simulink model "Planta_Funcional_17_03_24"  (R2021a)
settings: Solver=VariableStepAuto  StartTime=0.0  StopTime=120  MaxStep=1e-2  RelTol=1e-3
values from neighbouring files (symbols this model uses):
  ahmax = 0.75    [valoresPlanta_29_9_24.m]    (also in valoresPlanta_V3.m)
  alfahmax = ((2*ahmax)/(rhd))    (= 2)    [valoresPlanta_29_9_24.m]    (also in valoresPlanta_V3.m)
  alfatmax = atmax/rtd    (= 1.6)    [valoresPlanta_29_9_24.m]    (also in valoresPlanta_V3.m)
  atmax = 0.8    [valoresPlanta_29_9_24.m]    (also in valoresPlanta_V3.m)
  ax_max = 0.8    [valoresPlanta_29_9_24.m]    (also in valoresPlanta_v4.m)
  ay_max = 0.75    [valoresPlanta_29_9_24.m]    (also in valoresPlanta_v4.m)
  bcx = 1e6    (= 1000000)    [Valores_1.m]    (also in valoresPlanta.m; valoresPlanta_29_9_24.m; valoresPlanta_V3.m; valoresPlanta_v4.m)
  bcy = 1e7    (= 10000000)    [Valores_1.m]    (also in valoresPlanta.m; valoresPlanta_29_9_24.m; valoresPlanta_V3.m; valoresPlanta_v4.m)
  bh_eq = bhm*ih^2+bhd    (= 8720)    [Valores.m]    (also in Valores_1.m; valoresPlanta.m; valoresPlanta_29_9_24.m; valoresPlanta_V3.m)
  bhb = 1e8    (= 100000000)    [Valores.m]    (also in Valores_1.m; valoresPlanta.m; valoresPlanta_29_9_24.m; valoresPlanta_V3.m)
  bhEb = 2.2e9    (= 2200000000)    [Valores.m]    (also in Valores_1.m; valoresPlanta.m; valoresPlanta_29_9_24.m; valoresPlanta_V3.m)
  bt = 90.0    (= 90)    [Valores.m]    (also in Valores_1.m; valoresPlanta.m; valoresPlanta_29_9_24.m; valoresPlanta_V3.m)
  bt_eq = btd+(btm*(it^2))    (= 5401.8)    [valoresPlanta.m]    (also in valoresPlanta_29_9_24.m; valoresPlanta_V3.m; valoresPlanta_v4.m)
  btb = 5e6    (= 5000000)    [Valores.m]    (also in Valores_1.m; valoresPlanta.m; valoresPlanta_29_9_24.m; valoresPlanta_V3.m)
  btw = 3.0e3    (= 3000)    [Valores.m]    (also in Valores_1.m; valoresPlanta.m; valoresPlanta_29_9_24.m; valoresPlanta_V3.m)
  bwu = 150    [Valores.m]    (also in Valores_1.m; valoresPlanta.m; valoresPlanta_29_9_24.m; valoresPlanta_V3.m)
  estado_cont = [x_positions; hy_cont]    [perfilObsaculos.m]    (also in valoresPlanta_29_9_24.m = [x_positions; [hy_muelle hy_cont]])
  g = 9.80665    [Valores.m]    (also in Valores_1.m; valoresPlanta.m; valoresPlanta_29_9_24.m; valoresPlanta_V3.m)
  Hc = 0    [Valores.m]    (also in Valores_1.m = 2.5; valoresPlanta.m = 2.5; valoresPlanta_29_9_24.m = 2.5; valoresPlanta_V3.m = 2.5)
  hx_cont = 2.5    [perfilObsaculos.m]    (also in puntosTrayectoria.m; valoresPlanta_29_9_24.m)
  ih = 22    [Valores.m]    (also in Valores_1.m; valoresPlanta.m; valoresPlanta_29_9_24.m; valoresPlanta_V3.m)
  it = 30    [Valores.m]    (also in Valores_1.m; valoresPlanta.m; valoresPlanta_29_9_24.m; valoresPlanta_V3.m)
  Jh_eq = Jhm_hb*ih^2+Jhd_hEb    (= 18320)    [Valores.m]    (also in Valores_1.m; valoresPlanta.m; valoresPlanta_29_9_24.m; valoresPlanta_V3.m)
  Jt_eq = Jtd+(Jtm_tb*(it^2))    (= 7500)    [valoresPlanta.m]    (also in valoresPlanta_29_9_24.m; valoresPlanta_V3.m; valoresPlanta_v4.m)
  kcy = 1.8e9    (= 1800000000)    [Valores_1.m]    (also in valoresPlanta.m; valoresPlanta_29_9_24.m; valoresPlanta_V3.m; valoresPlanta_v4.m)
  KDh = Jeq2 * w_posh^3    (= -12245.4404091)    [Valores.m]    (also in Valores_1.m = Jeq2 * w_posh; valoresPlanta.m = Jeq2 * w_posh; valoresPlanta_29_9_24.m = Jh_eq * n * w_posh; valoresPlanta_V3.m = Jeq2 * w_posh)
  KDt = Meq2 * w_post^3    (= -4728.86946035)    [Valores.m]    (also in Valores_1.m = Meq2 * w_post; valoresPlanta.m = Meq2 * w_post; valoresPlanta_29_9_24.m = 10127; valoresPlanta_V3.m = Meq2 * w_post)
  KIh = Jeq2 * w_posh^2    (= 2572.66592082)    [Valores.m]    (also in Valores_1.m = Jeq2 * w_posh^3; valoresPlanta.m = Jeq2 * w_posh^3; valoresPlanta_29_9_24.m = Jh_eq * w_posh^3; valoresPlanta_V3.m = Jeq2 * w_posh^3)
  KIt = Meq2 * w_post^2    (= 1307.690244)    [Valores.m]    (also in Valores_1.m = Meq2 * w_post^3; valoresPlanta.m = Meq2 * w_post^3; valoresPlanta_29_9_24.m = 6809.6; valoresPlanta_V3.m = Meq2 * w_post^3)
  KPh = Jeq2 * w_posh    (= -540.495867769)    [Valores.m]    (also in Valores_1.m = Jeq2 * w_posh^2; valoresPlanta.m = Jeq2 * w_posh^2; valoresPlanta_29_9_24.m = Jh_eq * n * w_posh^2; valoresPlanta_V3.m = Jeq2 * w_posh^2)
  KPt = Meq2 * w_post    (= -361.62)    [Valores.m]    (also in Valores_1.m = Meq2 * w_post^2; valoresPlanta.m = Meq2 * w_post^2; valoresPlanta_29_9_24.m = 14123; valoresPlanta_V3.m = Meq2 * w_post^2)
  Ktw = 4.8e5    (= 480000)    [Valores.m]    (also in Valores_1.m; valoresPlanta.m; valoresPlanta_29_9_24.m; valoresPlanta_V3.m)
  kwu = 2.36e8    (= 236000000)    [Valores.m]    (also in Valores_1.m; valoresPlanta.m; valoresPlanta_29_9_24.m; valoresPlanta_V3.m)
  Mc_max = 5e4    (= 50000)    [Valores.m]    (also in Valores_1.m; valoresPlanta.m; valoresPlanta_29_9_24.m; valoresPlanta_V3.m)
  Mc_min = 2e3    (= 2000)    [Valores.m]    (also in Valores_1.m; valoresPlanta.m; valoresPlanta_29_9_24.m; valoresPlanta_V3.m)
  Meq = Mt+(it^2*Jtm_tb+Jtd)/rtd^2    (= 60000)    [Valores.m]    (also in Valores_1.m; valoresPlanta_29_9_24.m; valoresPlanta_v4.m)
  Mt = 30000    [Valores.m]    (also in Valores_1.m; valoresPlanta.m; valoresPlanta_29_9_24.m; valoresPlanta_V3.m)
  pos = [p0; p1; p2; p3; p4; p5]    [calcularTrayectoria2_prueba.m]    (also in perfilObsaculos.m = puntosTrayectoria(4, 1.5, 20, [-20,0], estado_cont, hy_cont,; puntosTrayectoria.m; valoresPlanta_29_9_24.m = calcularTrayectoria2_prueba(vx_max, vhmax, ax_max, Hc, hx_co)
  rhd = 0.75    [Valores.m]    (also in Valores_1.m; valoresPlanta.m; valoresPlanta_29_9_24.m; valoresPlanta_V3.m)
  rtd = 0.5    [Valores.m]    (also in Valores_1.m; valoresPlanta.m; valoresPlanta_29_9_24.m; valoresPlanta_V3.m)
  tau_hm = 1e-3    (= 0.001)    [valoresPlanta.m]    (also in valoresPlanta_29_9_24.m; valoresPlanta_V3.m; valoresPlanta_v4.m)
  tau_tm = 1e-3    (= 0.001)    [Valores.m]    (also in Valores_1.m; valoresPlanta.m; valoresPlanta_29_9_24.m; valoresPlanta_V3.m)
  Thb_Max = 5e4    (= 50000)    [Valores.m]    (also in Valores_1.m; valoresPlanta.m; valoresPlanta_29_9_24.m; valoresPlanta_V3.m)
  ThEb_Max = 1.1e6    (= 1100000)    [Valores.m]    (also in Valores_1.m; valoresPlanta.m; valoresPlanta_29_9_24.m; valoresPlanta_V3.m)
  Thm_Max = 2e4    (= 20000)    [Valores.m]    (also in Valores_1.m; valoresPlanta.m; valoresPlanta_29_9_24.m; valoresPlanta_V3.m)
  Ttb_Max = 5e3    (= 5000)    [Valores.m]    (also in Valores_1.m; valoresPlanta.m; valoresPlanta_29_9_24.m; valoresPlanta_V3.m)
  Ttm_Max = 3e3    (= 3000)    [Valores.m]    (also in Valores_1.m; valoresPlanta.m; valoresPlanta_29_9_24.m = 4000; valoresPlanta_V3.m)
  v_x_max = 4    [Valores_1.m]    (also in valoresPlanta.m; valoresPlanta_V3.m = 0.4; valoresPlanta_v4.m)
  vhmax = 3    [valoresPlanta_29_9_24.m]    (also in valoresPlanta_V3.m)
  vx_max = 4    [valoresPlanta_29_9_24.m]
  whmMax = P/Thm_Max    (= 47.8075)    [Valores_1.m]    (also in valoresPlanta.m; valoresPlanta_29_9_24.m = 176; valoresPlanta_V3.m; valoresPlanta_v4.m)
  wtmMax = (4/rtd)*it    (= 240)    [Valores_1.m]    (also in valoresPlanta.m; valoresPlanta_29_9_24.m; valoresPlanta_V3.m; valoresPlanta_v4.m)
  y0 = 2.5    [valoresPlanta_29_9_24.m]
  Yt0 = 45    [Valores.m]    (also in Valores_1.m; valoresPlanta.m; valoresPlanta_29_9_24.m; valoresPlanta_V3.m)
undefined symbols (not defined in the file or in its folder): sigbuilder_block, x0
libraries: vrlib x2, simulink_extras x1, aerolibanimutils x1, cstblocks x1, simulink x1
(part 1 of 2)
settings Model: Creator=Matias  LastModifiedBy=Matias

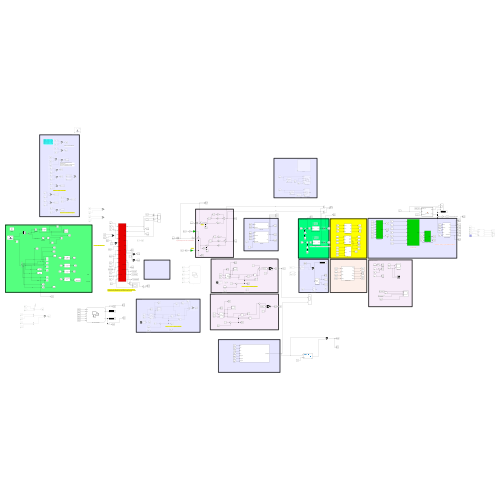
[thumbnail: Simulink's stored preview of the top-level diagram]
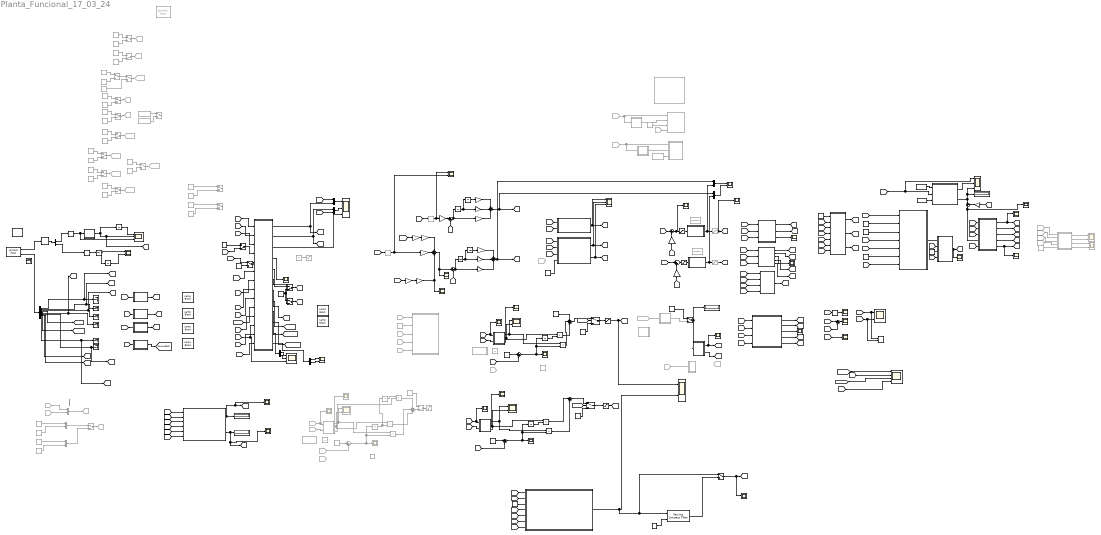
== system Planta_Funcional_17_03_24 ==
  note: Aca hacer la estimacion de masa
  note: Corregir con nivel 0 el estado de emergencia
  note: Estimación de carga: subir la carga lento (cuasiestático) y una vez que el cable esté completamente elongado determinar la masa. Se puede calcular para cierta velocidad cuanto debo demorar y darle ese tiempo para calcular la masa con la Fhw.
  note: FRENOS: 0 activados, 1 desactivados
  note: Frenos
  note: saturador a la salida?? o a la entrada de consigna de torque??
  note: Indicadores
  note: ciclo=0 y to_where=0 --> a barco
      | ciclo=0 y to_where=1 --> a muelle
      | -------------------------------------------------
      | ciclo=1 y to_where=0 --> a barco
      | ciclo=1 y to_where=1 --> a barco 2
      | ciclo=1 y to_where=2 --> a muelle
  note: revisar para modo manual
  note: ec2 cable tensado
  note: PI balanceo
  note: con ganancia baja, si sumo o resto no hace diferencia
  note: Control P
  note: por que v y no theta? no cambian las ganancias?
  note: d(theta)/dt
  note: Analisis de posiciones
  note: PD Balanceo
  note: Masa Variable
  note: Control Frenos
  note: Izaje
  note: Modulador de Torque
  note: Carro
  note: Movimiento
  note: PID Balanceo
  note: por que v y no theta? no cambian las ganancias?
  note: Control P
  note: valores de fila 1 de array son puntos medios de contenedores
  note: valor inicial, luego debe variar como
      | parametro local
      | cuando esta comentado: es parametro local
      | cuando no: es parametro de entrada
  note: debe venir de modo twistlocks
  note: HMI
  In4 : Inport
  BRKhE : Constant  Commented=on
  Balanceo : Scope
  Cable izaje elástico amortiguado : Subsystem
  Calculo theta,l y dl : Subsystem
  Carga Suspendida : Subsystem
  Chart : Stateflow chart  Commented=on  TreatAsAtomicUnit=on
  Chart1 : Stateflow chart  TreatAsAtomicUnit=on
  Chart2 : Stateflow chart  Commented=on  TreatAsAtomicUnit=on
  Chart3 : Stateflow chart  TreatAsAtomicUnit=on
  Chart4 : Stateflow chart  Commented=on  TreatAsAtomicUnit=on
  Chart5 : Stateflow chart  TreatAsAtomicUnit=on
  Chart6 : Stateflow chart  TreatAsAtomicUnit=on
  Chart7 : Stateflow chart  TreatAsAtomicUnit=on
  Chart8 : Stateflow chart  TreatAsAtomicUnit=on
  Chart9 : Stateflow chart  TreatAsAtomicUnit=on
  Constant{,15,17,20,42} (5 alike) : Constant  Value=0
  Constant1 : Constant  Value=65000
  Constant10 : Constant  Value=.8
  Constant{11,14,19,27,30,33,35,37,40,48} (10 alike) : Constant  Commented=on
  Constant12 : Constant  Commented=on  Value=45
  Constant{13,16,18,21,28..29,34,36,38..39,41,51} (12 alike) : Constant  Commented=on  Value=0
  Constant{2,5..6,9} (4 alike) : Constant  Value=Yt0
  Constant22 : Constant  Value=hx_cont
  Constant23 : Constant  Value=estado_cont
  Constant24 : Constant  Commented=on  Value=[-20 2.5 30 30]
  Constant25 : Constant  Commented=on  Value=[30 30 -10 5]
  Constant26 : Constant  Commented=on  Value=-10
  Constant3 : Constant  Value=kwu
  Constant31 : Constant  Commented=on  Value=2
  Constant{32,44..46} (4 alike) : Constant  Commented=on  Value=30
  Constant4 : Constant  Value=bwu
  Constant43 : Constant  Commented=on  Value=-10
  Constant47 : Constant  Commented=on  Value=5
  Constant49 : Constant  Commented=on  Value=-10
  Constant50 : Constant  Commented=on  Value=5
  Constant53 : Constant
  Constant54 : Constant  Value=30
  Constant55 : Constant  Value=30
  Constant7 : Constant  Commented=on  Value=Ttb_Max
  Constant8 : Constant
  Control Supervisor : Subsystem
  Controles : Subsystem  Commented=on
  Demux : Demux  Outputs=10
  Demux1 : Demux  Outputs=2
  Demux2 : Demux  Outputs=2
  Demux3 : Demux  Outputs=2
  Derivative : Derivative  Commented=on
  Derivative1 : Derivative  Commented=on
  Display{,1..3} (4 alike) : Display
  Enclavamiento carro : Stateflow chart  Commented=on  TreatAsAtomicUnit=on
  Enclavamiento izaje : Stateflow chart  Commented=on  TreatAsAtomicUnit=on
  Estimacion de Masa : Subsystem  Commented=on
  Fhw : Subsystem
  Freno Izaje : Subsystem
  Freno carro : Subsystem
  "Frenos Izaje " : Stateflow chart  Commented=on  TreatAsAtomicUnit=on
  Frenos Traslación : Stateflow chart  Commented=on  TreatAsAtomicUnit=on
  From100 : From  Commented=on  GotoTag=Fhw
  From103 : From  Commented=on  GotoTag=xl
  From104 : From  Commented=on  GotoTag=yl
  From27 : From  Commented=on  GotoTag=whm
  From28 : From  Commented=on  GotoTag=wtm
  From30 : From  Commented=on  GotoTag=whd
  From51 : From  Commented=on  GotoTag=xl
  From52 : From  Commented=on  GotoTag=xt
  From53 : From  Commented=on  GotoTag=hc
  From54 : From  Commented=on  GotoTag=yl
  From65 : From  Commented=on  GotoTag=tw
  From68 : From  Commented=on  GotoTag=theta
  From69 : From  Commented=on  GotoTag=l
  From70 : From  Commented=on  GotoTag=ml
  From71 : From  Commented=on  GotoTag=dTheta
  From72 : From  Commented=on  GotoTag=theta
  From80 : From  Commented=on  GotoTag=theta
  From81 : From  Commented=on  GotoTag=Fhw
  From82 : From  Commented=on  GotoTag=ml
  From83 : From  Commented=on  GotoTag=hc
  From95 : From  Commented=on  GotoTag=P_BEH
  Ftw : Subsystem
  Gain : Gain  Gain=bh_eq
  Gain1 : Gain  Gain=bt_eq
  Gain10 : Gain  Gain=1/rtd
  Gain11 : Gain  Gain=.01
  Gain12 : Gain  Gain=.01
  Gain13 : Gain  Gain=1/rtd
  Gain15 : Gain
  Gain2 : Gain  Gain=KIt
  Gain3 : Gain  Gain=KDh
  Gain4 : Gain  Gain=KPh
  Gain5 : Gain  Gain=KIh
  Gain6 : Gain  Gain=KPt
  Gain7 : Gain  Gain=KDt
  Gain8 : Gain  Gain=1/rtd
  Gain9 : Gain  Gain=2/rhd
  Goto23 : Goto  Commented=on  GotoTag=mr
  Goto28 : Goto  Commented=on  GotoTag=tw
  Goto30 : Goto  Commented=on  GotoTag=ciclo
  Goto31 : Goto  Commented=on  GotoTag=to_where
  Goto32 : Goto  Commented=on  GotoTag=START
  Goto33 : Goto  Commented=on  GotoTag=AUTO
  Goto34 : Goto  Commented=on  GotoTag=BALANCEO
  Goto37 : Goto  Commented=on  GotoTag=P_TB
  Goto38 : Goto  Commented=on  GotoTag=P_BH
  Goto39 : Goto  Commented=on  GotoTag=P_BEH
  Goto44 : Goto  Commented=on  GotoTag=p0
  Goto45 : Goto  Commented=on  GotoTag=p1
  Goto47 : Goto  Commented=on  GotoTag=S_TLK
  Integrator{,1..3,5..6,12..13} (8 alike) : Integrator
  Integrator{4,7,9..11} (5 alike) : Integrator  Commented=on
  Integrator8 : Integrator  InitialCondition=[0]  LimitOutput=on  UpperSaturationLimit=[3.5]  LowerSaturationLimit=[-3.5]
  Joystick 0 Tolerance1 : DeadZone  LowerValue=-0.3  UpperValue=0.3  SaturateOnIntegerOverflow=on
  Joystick 0 Tolerance2 : DeadZone  LowerValue=-0.2  UpperValue=0.2  SaturateOnIntegerOverflow=on
  Joystick Input : vrlib/Joystick Input  Commented=on  joyid=1  adjustports=on  forcefeed=off
  Joystick Input1 : vrlib/Joystick Input  joyid=1  adjustports=on  forcefeed=off
  Lamp : LampBlock
  Lamp1 : LampBlock
  MATLAB Function : MATLAB Function  TreatAsAtomicUnit=on
  Manual Switch{,2,5,20} (4 alike) : ManualSwitch
  Manual Switch1 : ManualSwitch  CurrentSetting=0
  Manual Switch{4,6..7,9..12,14..19} (13 alike) : ManualSwitch  Commented=on
  Manual Switch13 : ManualSwitch  Commented=on  CurrentSetting=0
  Manual Switch21 : ManualSwitch  CurrentSetting=0
  Manual Switch3 : ManualSwitch  Commented=on  CurrentSetting=0
  Manual Switch8 : ManualSwitch  Commented=on  CurrentSetting=0
  Modo Automatico : LampBlock  LabelPosition=Hide
  Modo Twistlocks : Stateflow chart  TreatAsAtomicUnit=on
  Modulador de Torque Carro : Subsystem
  Modulador de Torque Izaje : Subsystem
  Mux{,1..3} (4 alike) : Mux  Inputs=2
  Mux6 : Mux  Commented=on  Inputs=2
  Product{,1..2,6} (4 alike) : Product
  Product3 : Product  Commented=on
  Product4 : Product  Commented=on
  Product5 : Product  Commented=on
  Radians to Degrees : simulink_extras/Transformations/Radians to Degrees
  Rate Limiter1 : RateLimiter  Commented=through  RisingSlewLimit=ay_max  FallingSlewLimit=-ay_max  SampleTimeMode=inherited
  Rate Limiter2 : RateLimiter  Commented=through  RisingSlewLimit=ax_max  FallingSlewLimit=-ax_max  SampleTimeMode=inherited
  START : LampBlock  LabelPosition=Hide
  Saturation : Saturate  Commented=through  UpperLimit=Thm_Max  LowerLimit=-Thm_Max
  Saturation1 : Saturate  Commented=through  UpperLimit=Ttm_Max  LowerLimit=-Ttm_Max
  Saturation2 : Saturate  UpperLimit=4  LowerLimit=-4
  Saturation3 : Saturate  Commented=on  UpperLimit=v_x_max  LowerLimit=-4
  Saturation4 : Saturate  Commented=on  UpperLimit=4  LowerLimit=-4
  Saturation5 : Saturate  UpperLimit=4  LowerLimit=-4
  Saturation6 : Saturate  UpperLimit=Ttm_Max  LowerLimit=-Ttm_Max
  Saturation7 : Saturate  UpperLimit=Thm_Max  LowerLimit=-Thm_Max
  Scope{,4,6,8..10,12..14,19,21..23,25..26,28..30,32,35..36} (21 alike) : Scope
  Scope{1..2,5,7,20,34,38} (7 alike) : Scope  NumInputPorts=2
  Scope11 : Scope  Commented=on  NumInputPorts=2
  Scope15 : Scope  Commented=on
  Scope16 : Scope  Commented=on  NumInputPorts=2
  Scope17 : Scope  Commented=on
  Scope18 : Scope  Commented=on
  Scope{3,24,31,33,37} (5 alike) : Scope  NumInputPorts=3
  Scope27 : Scope  Commented=on  NumInputPorts=2
  Selector : Selector  InputPortWidth=5  IndexOptions=Index vector (dialog)  Indices=[1 4]  OutputSizes=1
  Seteo punto de llegada : Stateflow chart  TreatAsAtomicUnit=on
  Simulation Pace : aerolibanimutils/Simulation Pace  SimulationPace=1  SleepMode=Auto  OutputPaceError=off  SampleTime=1/50
  Subsistema Carro : Subsystem
  Subsistema Izaje : Subsystem
  Subsistema Tambor : Subsystem
  Subsystem : Subsystem
  Subsystem2 : Subsystem  Commented=on
  Sum : Sum  Inputs=|++
  Sum{1,4,6,9,12,15} (6 alike) : Sum  Inputs=|+-
  Sum10 : Sum  Commented=on  Inputs=|+-
  Sum11 : Sum  Commented=on  Inputs=+++
  Sum13 : Sum  Inputs=|++
  Sum2 : Sum  Inputs=+++
  Sum3 : Sum  Inputs=|++
  Sum5 : Sum  Inputs=+++
  Sum7 : Sum  Inputs=+++
  Sum8 : Sum  Inputs=-++
  Switch : Switch  Criteria=u2 > Threshold
  Switch1 : Switch  Criteria=u2 > Threshold
  TWISLOCK : LampBlock  LabelPosition=Hide
  Terminator{,1..6} (7 alike) : Terminator
  Transfer Fcn : TransferFcn  Commented=on  Denominator=[1e-3 1]
  Transfer Fcn1 : TransferFcn  Commented=on  Denominator=[1e-3 1]
  Varying Lowpass Filter : cstblocks/Linear Parameter Varying/Varying Lowpass Filter  N=1
  Vector Concatenate1 : Concatenate  Commented=on  Mode=Multidimensional array  ConcatenateDimension=2
  Vector Concatenate2 : Concatenate  Commented=on  Mode=Multidimensional array  ConcatenateDimension=2
  Vector Concatenate3 : Concatenate  Commented=on  Mode=Multidimensional array  ConcatenateDimension=2
  XY Graph : simulink/Sinks/XY Graph  xmin=-1  xmax=1  ymin=-1  ymax=1  st=-1
  at(t) : Scope
  atd(t) : Scope
  graficos : Stateflow chart  Commented=on  TreatAsAtomicUnit=on
  modo doble : LampBlock  LabelPosition=Hide
  posicion : Scope  NumInputPorts=2
  posicion1 : Scope  NumInputPorts=4
  whd*(t)1 : Subsystem  Tag=STV Subsys  Commented=on  LoadFcn=sigbuilder_block('load');  StartFcn=sigbuilder_block('start');  StopFcn=sigbuilder_block('stop');  ClipboardFcn=sigbuilder_block('clipboard');  mask(Sigbuilder block){tuvar=[0:10]}
      mask help: Simulink:masks:SigbuilderBlock_MD
      mask init:
      | if ~strcmp(get_param(bdroot(gcbh),'SimulationStatus'),'stopped') tuvar = sigbuilder_block('maskInit'); end
      settings: CopyFcn=sigbuilder_block('copy');  DeleteFcn=sigbuilder_block('delete');  ModelCloseFcn=sigbuilder_block('modelClose');  PreSaveFcn=sigbuilder_block('preSave');  PauseFcn=sigbuilder_block('pause');  ContinueFcn=sigbuilder_block('continue');  NameChangeFcn=sigbuilder_block('namechange');  OpenFcn=sigbuilder_block('open',[437.6 199.2 550.4 400 ]);  CloseFcn=sigbuilder_block('close');
      mask Display: plot(0, 0, 100, 100,[2, 2, 32, 32, 2], [68, 8, 8, 68, 68],[32, 2], [38, 38], [32, 19, 2],[53, 60, 44], [32, 17, 17, 2],[16, 16, 31, 31]);txt = getActiveGroup(gcbh);text(2, 100, txt,'verticalAlignment', 'top');
  whd*(t)2 : Subsystem  Tag=STV Subsys  Commented=on  LoadFcn=sigbuilder_block('load');  StartFcn=sigbuilder_block('start');  StopFcn=sigbuilder_block('stop');  ClipboardFcn=sigbuilder_block('clipboard');  mask(Sigbuilder block){tuvar=[0:10]}
      mask help: Simulink:masks:SigbuilderBlock_MD
      mask init:
      | if ~strcmp(get_param(bdroot(gcbh),'SimulationStatus'),'stopped') tuvar = sigbuilder_block('maskInit'); end
      settings: CopyFcn=sigbuilder_block('copy');  DeleteFcn=sigbuilder_block('delete');  ModelCloseFcn=sigbuilder_block('modelClose');  PreSaveFcn=sigbuilder_block('preSave');  PauseFcn=sigbuilder_block('pause');  ContinueFcn=sigbuilder_block('continue');  NameChangeFcn=sigbuilder_block('namechange');  OpenFcn=sigbuilder_block('open',[437.6 199.2 550.4 400 ]);  CloseFcn=sigbuilder_block('close');
      mask Display: plot(0, 0, 100, 100,[2, 2, 32, 32, 2], [68, 8, 8, 68, 68],[32, 2], [38, 38], [32, 19, 2],[53, 60, 44], [32, 17, 17, 2],[16, 16, 31, 31]);txt = getActiveGroup(gcbh);text(2, 100, txt,'verticalAlignment', 'top');
  x carro : Scope
  wires:
  Subsistema Tambor/1(xtd(t)) -> [xtd]
  Subsistema Tambor/2(vtd(t)) -> [vtd]
  Subsistema Carro/1(xt(t)) -> [xt]
  Subsistema Carro/2(vt(t)) -> [vt]
  Subsistema Carro/3(at(t)) -> at(t)/1
  Subsistema Tambor/3(atd(t)) -> atd(t)/1
  [Ttb] -> Subsistema Tambor/2(Ttb(t))
  [Ttm] -> Subsistema Tambor/1(Tm(t))
  [Ftw] -> Subsistema Carro/3(Ftw(t))
  [Fhw] -> Subsistema Carro/2(Fhw(t))
  [theta] -> Subsistema Carro/1(theta(t))
  [Ftw] -> Subsistema Tambor/3(Ftw(t))
  Ftw/1(Ftw(t)) -> [Ftw]
  [xtd] -> Ftw/1(xtd(t))
  [xt] -> Ftw/2(xt(t))
  [vtd] -> Ftw/3(vtd(t))
  [vt] -> Ftw/4(vt(t))
  [Thm] -> Subsistema Izaje/2(Thm(t))
  [Thb] -> Subsistema Izaje/1(Thb(t))
  [Fhw] -> Subsistema Izaje/3(Fhw(t))
  Subsistema Izaje/1(xh(t)) -> [xh]
  Subsistema Izaje/2(vh(t)) -> [vh]
  Subsistema Izaje/3(ah(t)) -> Scope/1
  Subsistema Izaje/4(whm(t)) -> [whm]
  Subsistema Tambor/4(wtm(t)) -> [wtm]
  [dxl] -> Calculo theta,l y dl/5(dxl)
  Constant2/1 -> Calculo theta,l y dl/1(Yt0)
  [yl] -> Calculo theta,l y dl/2(yl)
  Calculo theta,l y dl/3(dl) -> [dl]
  Calculo theta,l y dl/1(l) -> [l]
  [dyl] -> Calculo theta,l y dl/7(dyl)
  [xl] -> Calculo theta,l y dl/3(xl)
  [vt] -> Calculo theta,l y dl/6(vt)
  [xt] -> Calculo theta,l y dl/4(xt)
  Calculo theta,l y dl/2(theta) -> [theta]
  [dl] -> Fhw/4(dl(t))
  [xh] -> Fhw/7(xh(t))
  Constant3/1 -> Fhw/2(kwu)
  [l] -> Fhw/1(l(t))
  Constant5/1 -> Fhw/6(Yt0)
  [vh] -> Fhw/5(vh(t))
  Constant4/1 -> Fhw/3(bwu)
  Fhw/1(Fhw(t)) -> Cable izaje elástico amortiguado/1(Fhw)
  [l] -> Cable izaje elástico amortiguado/2(l(t))
  Constant6/1 -> Cable izaje elástico amortiguado/3(Yt0)
  [xh] -> Cable izaje elástico amortiguado/4(xh(t))
  Cable izaje elástico amortiguado/1(Fhw(t)) -> Scope14/1, [Fhw]
  [theta] -> Carga Suspendida/2(theta(t))
  [Fhw] -> Carga Suspendida/1(Fhw(t))
  Carga Suspendida/1(xl(t)) -> Scope23/1, [xl]
  Carga Suspendida/4(dyl(t)) -> [dyl]
  Carga Suspendida/3(yl(t)) -> [yl]
  Carga Suspendida/2(dxl(t)) -> [dxl]
  From27/1 -> "Frenos Izaje "/1(whm), Enclavamiento izaje/1(whm)
  From28/1 -> Enclavamiento carro/1(wtm), Frenos Traslación/1(wtm)
  Enclavamiento carro/1(BRKt) -> Frenos Traslación/2(BRKt)
  Enclavamiento izaje/1(BRKh) -> "Frenos Izaje "/2(BRKh)
  Constant7/1 -> Frenos Traslación/3(Ttb_Max)
  BRKhE/1 -> "Frenos Izaje "/3(BRKhE)
  Subsistema Izaje/5(whd(t)) -> [whd]
  [ThEb] -> Subsistema Izaje/4(ThEb(t))
  From30/1 -> "Frenos Izaje "/4(whd)
  [Thm_] -> Sum/1
  Sum/1 -> Saturation7/1
  [whd] -> Gain/1
  Gain/1 -> Sum/2
  Integrator1/1 -> Gain5/1
  Integrator/1 -> Integrator1/1, Gain4/1
  Sum1/1 -> Integrator/1, Gain3/1
  Gain4/1 -> Sum2/2
  Gain5/1 -> Sum2/1
  Gain3/1 -> Sum2/3
  Sum3/1 -> Scope29/1, Saturation6/1
  [Ttm_] -> Sum3/1
  Gain1/1 -> Sum3/2
  Subsistema Tambor/5(wtd(t)) -> [wtd]
  [wtd] -> Gain1/1
  Gain7/1 -> Sum5/3
  [wtd] -> Sum4/2
  Gain6/1 -> Sum5/2
  Gain2/1 -> Sum5/1
  Integrator2/1 -> Integrator3/1, Gain6/1
  Sum4/1 -> Gain7/1, Integrator2/1
  Integrator3/1 -> Gain2/1
  [xl] -> XY Graph/1, posicion/1  "xl"
  [yl] -> XY Graph/2, posicion/2  "yl"
  [whd] -> Sum1/2
  [ml] -> Carga Suspendida/3(ml)
  [l] -> Scope8/1, Chart1/1(l)
  [ml] -> Chart1/2(ml)
  Product/1 -> Sum7/3
  Product1/1 -> Sum7/2
  Chart1/1(KD) -> Scope7/1, Product1/1
  Chart1/2(KP) -> Scope7/2, Product/1
  Constant/1 -> Sum6/1
  Sum8/1 -> Scope10/1, Sum4/1
  Sum7/1 -> Switch1/1
  Constant1/1 -> Manual Switch/1
  [yl] -> Control Supervisor/3(yl)
  Control Supervisor/2(vXref) -> [vXref], Mux1/1  "vXref"
  Control Supervisor/1(vYref) -> [vYref], Mux/2  "vYref"
  [xl] -> Control Supervisor/1(xl)
  Gain9/1 -> Sum1/1
  Constant12/1 -> graficos/2(Yt0)
  From52/1 -> graficos/4(xt)
  From51/1 -> graficos/3(xl)
  From53/1 -> graficos/1(Hc)
  From54/1 -> graficos/5(yl)
  [xl] -> Sum9/1
  [xt] -> Sum9/2
  Sum9/1 -> Scope6/1
  [xt] -> x carro/1
  Radians to Degrees/1 -> Balanceo/1
  [theta] -> Radians to Degrees/1
  Chart1/3(WN) -> Scope9/1
  Integrator5/1 -> Product/2
  Gain8/1 -> Gain11/1
  [Vxt_] -> Gain8/1
  Gain10/1 -> Sum8/2
  [xt] -> Control Supervisor/2(xt)
  [dyl] -> Subsystem/7(d(yl(t))/dt)
  [vt] -> Subsystem/6(d(xt(t))/dt)
  [dxl] -> Subsystem/5(d(xl(t))/dt)
  [yl] -> Subsystem/4(yl(t))
  [xt] -> Subsystem/2(xt(t))
  [xl] -> Subsystem/1(xl(t))
  Constant9/1 -> Subsystem/3(Yto)
  [vXref] -> Rate Limiter2/1  "vXref"
  [vYref] -> Rate Limiter1/1  "vYref"
  Sum2/1 -> [Thm_], Mux3/1  "Thm_"
  Sum5/1 -> [Ttm_], Mux2/1  "Ttm_"
  Switch1/1 -> Saturation2/1
  [dTheta] -> Sum6/2
  Saturation2/1 -> Scope1/1, [Vxt_]
  Rate Limiter1/1 -> Scope5/1, Gain9/1
  Rate Limiter2/1 -> Gain10/1, Scope5/2
  [vh] -> Mux/1
  [vt] -> Mux1/2
  Mux1/1 -> Scope3/2
  Mux/1 -> Scope3/1
  Subsystem/1(d(theta(t))/dt) -> Manual Switch2/1, Varying Lowpass Filter/1, Scope1/2
  Varying Lowpass Filter/1 -> Manual Switch2/2
  Constant10/1 -> Varying Lowpass Filter/2
  Manual Switch2/1 -> Scope12/1, [dTheta]
  Sum6/1 -> Scope13/1, Product1/2, Integrator5/1
  Mux2/1 -> Scope2/1
  Mux3/1 -> Scope2/2
  Integrator7/1 -> Saturation3/1  "vXref"
  Constant15/1 -> Sum7/1
  Chart2/4(KI) -> Product5/2
  Product3/1 -> Sum11/3
  Sum11/1 -> Manual Switch3/2
  Chart2/2(KP) -> Product3/1, Scope16/2
  Integrator11/1 -> Product5/1
  From71/1 -> Sum10/2
  Integrator10/1 -> Integrator11/1, Product3/2
  Chart2/3(WN) -> Scope18/1
  Constant18/1 -> Manual Switch3/1
  Constant16/1 -> Sum10/1
  Chart2/1(KD) -> Scope16/1, Product4/1
  From70/1 -> Chart2/2(ml)
  Product4/1 -> Sum11/2
  From69/1 -> Scope17/1, Chart2/1(l)
  Sum10/1 -> Scope15/1, Product4/2, Integrator10/1
  Manual Switch3/1 -> Saturation4/1
  Product5/1 -> Sum11/1
  [theta] -> Sum12/2
  Chart3/3(KI) -> Scope20/2, Product2/1
  [ml] -> Chart3/2(ml)
  [l] -> Scope21/1, Chart3/1(l)
  Switch/1 -> Saturation5/1
  Integrator12/1 -> Product2/2
  Chart3/2(WN) -> Scope22/1
  Sum12/1 -> Scope19/1, Product6/2, Integrator12/1
  Chart3/1(KP) -> Product6/1, Scope20/1
  Product6/1 -> Sum13/2
  Sum13/1 -> Switch/1
  Constant20/1 -> Switch/3
  Product2/1 -> Sum13/1
  Constant17/1 -> Sum12/1
  Saturation5/1 -> [Vx_PI]
  Gain12/1 -> Sum8/1
  Gain13/1 -> Gain12/1
  [Vx_PI] -> Gain13/1
  Modo Twistlocks/1(hc) -> Scope28/1, [hc]
  [hc] -> Carga Suspendida/5(hc)
  Constant22/1 -> MATLAB Function/3(anchoCont)
  Constant23/1 -> MATLAB Function/1(estado_cont)
  [xt] -> Scope24/1, MATLAB Function/2(xl)
  Gain15/1 -> Sum15/2
  [hc] -> Gain15/1
  MATLAB Function/1(index) -> Scope24/2
  Gain11/1 -> Scope4/1, Sum8/3
  Modulador de Torque Carro/1(Ttm(t)) -> Saturation1/1, Mux2/2
  Modulador de Torque Izaje/1(Thm(t)) -> Saturation/1, Mux3/2
  Saturation1/1 -> Scope26/1, [Ttm]
  Saturation/1 -> [Thm]
  From80/1 -> Subsystem2/1(Theta)
  From81/1 -> Subsystem2/2(Fhw1)
  From82/1 -> Subsystem2/3(ml)
  From83/1 -> Subsystem2/4(hc)
  Subsystem2/1(xl) -> Scope11/1
  Subsystem2/2(yl) -> Scope11/2
  Subsystem2/3(xl') -> Scope27/1
  Subsystem2/4(yl') -> Scope27/2
  MATLAB Function/2(y_evol) -> Display3/1, Scope24/3, Sum15/1
  Constant26/1 -> Subsystem2/5(yc0)
  Sum15/1 -> Carga Suspendida/4(yc0), Scope32/1
  Carga Suspendida/5(estadoContacto) -> Scope25/1, [eCon]
  Constant29/1 -> Manual Switch9/1
  Constant28/1 -> Manual Switch8/2
  Manual Switch8/1 -> Goto30/1
  Constant21/1 -> Manual Switch7/2
  Manual Switch9/1 -> Manual Switch10/1
  Manual Switch10/1 -> Goto31/1
  Constant27/1 -> Manual Switch8/1
  Manual Switch7/1 -> Goto28/1
  Constant30/1 -> Manual Switch9/2
  Constant19/1 -> Manual Switch7/1
  Constant31/1 -> Manual Switch10/2
  Control Supervisor/3(estado) -> Scope3/3
  Constant33/1 -> Manual Switch11/1
  Manual Switch11/1 -> Goto32/1
  Constant34/1 -> Manual Switch11/2
  [start1] -> Control Supervisor/7(START)
  Manual Switch12/1 -> Goto33/1
  Constant35/1 -> Manual Switch12/1
  Constant36/1 -> Manual Switch12/2
  Control Supervisor/4(FINISH) -> Scope30/1
  Saturation6/1 -> Modulador de Torque Carro/1(Ttm*(t))
  Saturation7/1 -> Modulador de Torque Izaje/1(Thm*(t))
  Constant38/1 -> Manual Switch13/2
  Constant37/1 -> Manual Switch13/1
  Manual Switch13/1 -> Goto34/1
  [M_BAL] -> Switch/2
  Freno Izaje/1(Thb) -> Scope31/2, [Thb]
  Freno Izaje/2(ThEb) -> Scope31/3, [ThEb]
  Freno carro/1(Ttb) -> Scope31/1, [Ttb]
  [whm] -> Freno Izaje/1(whm)
  [wtm] -> Freno carro/1(wtm)
  [whd] -> Freno Izaje/3(whd)
  Manual Switch4/1 -> Goto37/1
  Constant13/1 -> Manual Switch4/2
  Constant11/1 -> Manual Switch4/1
  Manual Switch14/1 -> Goto38/1
  Constant39/1 -> Manual Switch14/2
  Constant14/1 -> Manual Switch14/1
  Manual Switch15/1 -> Goto39/1
  Constant41/1 -> Manual Switch15/2
  Constant40/1 -> Manual Switch15/1
  [P_TB] -> Freno carro/2(pulsadorTb)
  [P_BH] -> Freno Izaje/2(pulsadorBh)
  [eCon] -> Control Supervisor/6(eCon)
  [wtm] -> Control Supervisor/9(wtm)
  [whm] -> Control Supervisor/8(whm)
  Control Supervisor/6(BRKt) -> Manual Switch5/2
  Control Supervisor/5(BRKh) -> Manual Switch1/1
  [BALANCEO] -> Control Supervisor/10(bBal)
  Control Supervisor/7(mBal) -> [M_BAL]
  [M_BAL] -> Switch1/2
  Constant42/1 -> Switch1/3
  Manual Switch1/1 -> [P_TB]
  Manual Switch5/1 -> [P_BH]
  Constant8/1 -> Manual Switch5/1, Manual Switch1/2
  From100/1 -> Estimacion de Masa/1(Fhw)
  [Fhw] -> Control Supervisor/11(Fhw)
  [AUTO] -> Scope37/3, Control Supervisor/12(In17)
  Constant24/1 -> Manual Switch6/1
  Constant25/1 -> Manual Switch6/2
  Constant50/1 -> Vector Concatenate1/2
  Constant49/1 -> Vector Concatenate1/1
  Constant46/1 -> Vector Concatenate2/2
  Constant45/1 -> Vector Concatenate2/1
  From103/1 -> Vector Concatenate3/1  "xl"
  From104/1 -> Vector Concatenate3/2
  Vector Concatenate3/1 -> Goto44/1
  Manual Switch16/1 -> Goto45/1
  Vector Concatenate1/1 -> Manual Switch16/2
  Vector Concatenate2/1 -> Manual Switch16/1
  Constant44/1 -> Manual Switch18/1
  Constant32/1 -> Manual Switch17/1
  Constant43/1 -> Manual Switch17/2
  Constant47/1 -> Manual Switch18/2
  Control Supervisor/8(tw) -> [modo_tw]
  From65/1 -> Chart/1(tw)
  Constant48/1 -> Manual Switch19/1
  Constant51/1 -> Manual Switch19/2
  Manual Switch19/1 -> Goto47/1
  Chart/1(Mcx) -> Manual Switch/2
  Modo Twistlocks/2(ml) -> [ml]
  [tw] -> Control Supervisor/13(Select_TLK)
  ? -> Terminator6/1
  Chart9/1(vyOut) -> [vyJoy], Scope33/2, Integrator6/1  "vy_conSensibilidad"
  Joystick 0 Tolerance2/1 -> Scope33/3, Chart9/1(vy)
  Integrator6/1 -> Scope33/1  "y"
  Chart7/1(start) -> [start1]
  Integrator13/1 -> Scope34/2  "y"
  Demux1/2 -> Joystick 0 Tolerance1/1  "vy_analog_der_hor"
  Chart8/1(modo) -> [BALANCEO]
  [botX] -> Seteo punto de llegada/5(X)
  Seteo punto de llegada/1(y) -> Scope36/1, [Yobj], Display1/1
  Joystick 0 Tolerance1/1 -> Integrator8/1
  Demux1/1 -> Joystick 0 Tolerance2/1  "vx_analog_izq_hor"
  [botA] -> Seteo punto de llegada/3(A)
  [back] -> Seteo punto de llegada/1(back)
  Selector/1 -> Demux1/1
  [botB] -> Seteo punto de llegada/6(B)
  Integrator8/1 -> Integrator13/1, Scope34/1  "vy"
  Demux/9 -> [L3]  "L3"
  Joystick Input1/2 -> Demux/1
  [botY] -> Seteo punto de llegada/4(Y)
  Joystick Input1/1 -> Selector/1
  Demux/8 -> [start], Terminator5/1  "START"
  Chart6/1(TWIS) -> [tw]
  [RB] -> Chart5/1(RB)
  Demux/5 -> [LB]  "LB"
  Demux/4 -> [botY], Terminator3/1  "Y"
  Demux/7 -> [back], Terminator4/1  "BACK"
  [L3] -> Chart7/1(L3)
  Demux/10 -> [R3]  "R3"
  Demux/3 -> [botX], Terminator2/1  "X"
  Demux/2 -> [botB], Terminator1/1  "B"
  Chart5/1(automatic) -> [AUTO]
  Demux/6 -> [RB]  "RB"
  Demux/1 -> [botA], Terminator/1  "A"
  [start] -> Seteo punto de llegada/2(start)
  [R3] -> Chart8/1(R3)
  [LB] -> Chart6/1(LB)
  Constant53/1 -> Freno Izaje/4(pulsadorBEh)
  Constant55/1 -> Manual Switch20/2
  [Yobj] -> Manual Switch20/1
  Manual Switch20/1 -> Control Supervisor/5(y_obj)
  [Xobj] -> Manual Switch21/2
  Constant54/1 -> Manual Switch21/1
  Manual Switch21/1 -> Control Supervisor/4(x_obj)
  Seteo punto de llegada/2(x) -> Scope35/1, [Xobj], Display2/1
  Manual Switch/1 -> Modo Twistlocks/1(Mcx), Display/1
  [vyJoy] -> Control Supervisor/14(vyJoy)
  [isFhwEstable] -> posicion1/3
  [ml_estimado] -> posicion1/1
  [Fhw] -> posicion1/4
  [ml] -> posicion1/2
  Control Supervisor/9(ml_estimado) -> [ml_estimado]
  Control Supervisor/10(isFhwEstable) -> [isFhwEstable]
  Control Supervisor/11(p0) -> Demux2/1
  Demux2/1 -> Scope37/1
  Demux2/2 -> Scope37/2
  Control Supervisor/12(p1) -> Demux3/1
  Demux3/1 -> Scope38/1
  Demux3/2 -> Scope38/2

== system Planta_Funcional_17_03_24/Cable izaje elástico amortiguado ==
  note: l_h
  Fhw : Inport
  l(t) : Inport  Port=2
  Yt0 : Inport  Port=3
  xh(t) : Inport  Port=4
  Constant9 : Constant  Value=0
  Relational Operator : RelationalOperator  OutDataTypeStr=boolean  RndMeth=Simplest
  Sum : Sum  Inputs=|+-
  Switch1 : Switch  Criteria=u2 > Threshold
  Fhw(t) : Outport
  wires:
  l(t)/1 -> Relational Operator/1
  Sum/1 -> Relational Operator/2
  Fhw/1 -> Switch1/1
  Yt0/1 -> Sum/1
  Constant9/1 -> Switch1/3
  Relational Operator/1 -> Switch1/2
  xh(t)/1 -> Sum/2
  Switch1/1 -> Fhw(t)/1

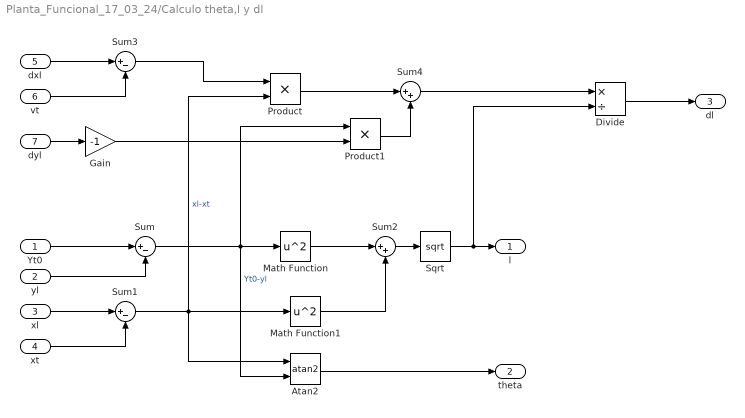
== system Planta_Funcional_17_03_24/Calculo theta,l y dl ==
  Yt0 : Inport
  yl : Inport  Port=2
  xl : Inport  Port=3
  xt : Inport  Port=4
  dxl : Inport  Port=5
  vt : Inport  Port=6
  dyl : Inport  Port=7
  Atan2 : Trigonometry  Operator=atan2
  Divide : Product  Inputs=*/
  Gain : Gain  Gain=-1
  Math Function : Math  Operator=square  SaturateOnIntegerOverflow=on
  Math Function1 : Math  Operator=square  SaturateOnIntegerOverflow=on
  Product : Product
  Product1 : Product
  Sqrt : Sqrt  SaturateOnIntegerOverflow=on
  Sum : Sum  Inputs=|+-
  Sum1 : Sum  Inputs=|+-
  Sum2 : Sum  Inputs=|++
  Sum3 : Sum  Inputs=|+-
  Sum4 : Sum  Inputs=|++
  l : Outport
  theta : Outport  Port=2
  dl : Outport  Port=3
  wires:
  Yt0/1 -> Sum/1
  yl/1 -> Sum/2
  xl/1 -> Sum1/1
  xt/1 -> Sum1/2
  Atan2/1 -> theta/1
  Sum1/1 -> Product/2, Math Function1/1, Atan2/1  "xl-xt"
  Sum/1 -> Product1/1, Atan2/2, Math Function/1  "Yt0-yl"
  Math Function/1 -> Sum2/1
  Math Function1/1 -> Sum2/2
  Sum2/1 -> Sqrt/1
  Sqrt/1 -> Divide/2, l/1
  dxl/1 -> Sum3/1
  vt/1 -> Sum3/2
  Sum3/1 -> Product/1
  dyl/1 -> Gain/1
  Gain/1 -> Product1/2
  Product/1 -> Sum4/1
  Product1/1 -> Sum4/2
  Sum4/1 -> Divide/1
  Divide/1 -> dl/1

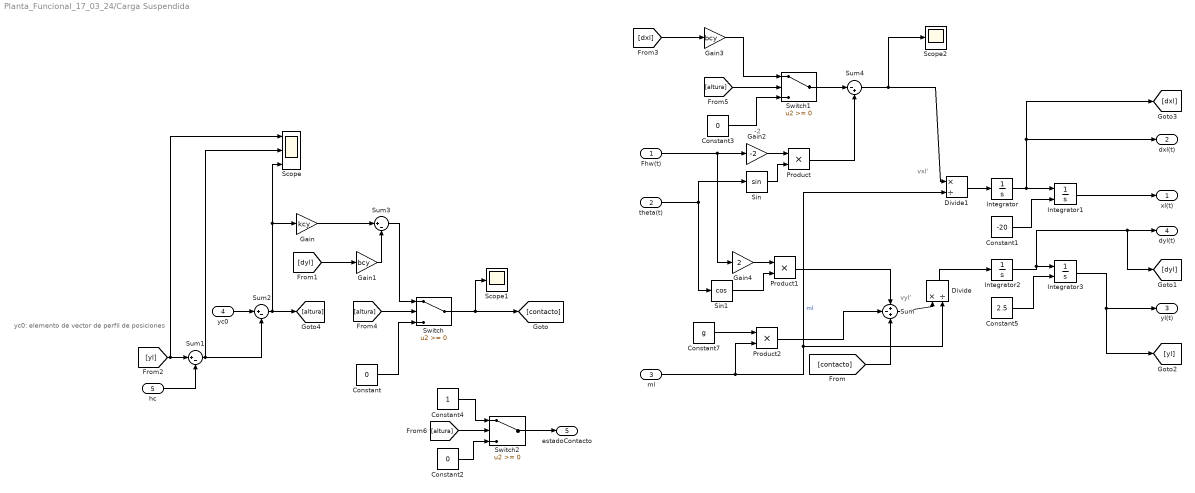
== system Planta_Funcional_17_03_24/Carga Suspendida ==
  note: -2
  note: vxl'
  note: vyl'
  note: yc0: elemento de vector de perfil de posiciones
  Fhw(t) : Inport
  theta(t) : Inport  Port=2
  ml : Inport  Port=3
  yc0 : Inport  Port=4
  hc : Inport  Port=5
  Constant : Constant  Value=0
  Constant1 : Constant  Value=-20
  Constant2 : Constant  Value=0
  Constant3 : Constant  Value=0
  Constant4 : Constant
  Constant5 : Constant  Value=2.5
  Constant7 : Constant  Value=g
  Divide : Product  Inputs=*/
  Divide1 : Product  Inputs=*/
  Gain : Gain  Gain=kcy
  Gain1 : Gain  Gain=bcy
  Gain2 : Gain  Gain=-2
  Gain3 : Gain  Gain=bcy
  Gain4 : Gain  Gain=2
  Integrator : Integrator
  Integrator1 : Integrator  InitialConditionSource=external
  Integrator2 : Integrator
  Integrator3 : Integrator  InitialConditionSource=external
  Product : Product
  Product1 : Product
  Product2 : Product
  Scope : Scope  NumInputPorts=3
  Scope1 : Scope
  Scope2 : Scope
  Sin : Trigonometry
  Sin1 : Trigonometry  Operator=cos
  Sum : Sum  Inputs=+-+
  Sum1 : Sum  Inputs=|+-
  Sum2 : Sum  Inputs=|+-
  Sum3 : Sum  Inputs=|+-
  Sum4 : Sum  Inputs=|-+
  Switch : Switch
  Switch1 : Switch
  Switch2 : Switch
  xl(t) : Outport
  dxl(t) : Outport  Port=2
  yl(t) : Outport  Port=3
  dyl(t) : Outport  Port=4
  estadoContacto : Outport  Port=5
  wires:
  Divide1/1 -> Integrator/1
  theta(t)/1 -> Sin1/1, Sin/1
  Constant7/1 -> Product2/1
  Product2/1 -> Sum/2
  Product/1 -> Sum4/2
  Fhw(t)/1 -> Gain4/1, Gain2/1
  Sum/1 -> Divide/1
  Integrator/1 -> [dxl], dxl(t)/1, Integrator1/1
  Sin1/1 -> Product1/2
  Gain2/1 -> Product/1
  Product1/1 -> Sum/1
  Sin/1 -> Product/2
  Integrator1/1 -> xl(t)/1
  Integrator2/1 -> [dyl], dyl(t)/1, Integrator3/1
  Divide/1 -> Integrator2/1
  Gain4/1 -> Product1/1
  Integrator3/1 -> [yl], yl(t)/1
  ml/1 -> Product2/2, Divide1/2, Divide/2  "ml"
  [yl] -> Scope/1, Sum1/1
  hc/1 -> Sum1/2
  Sum1/1 -> Scope/2, Sum2/2
  yc0/1 -> Sum2/1
  Constant/1 -> Switch/3
  [dyl] -> Gain1/1
  Gain1/1 -> Sum3/2
  Gain/1 -> Sum3/1
  Sum2/1 -> [altura], Scope/3, Gain/1
  Sum3/1 -> Switch/1
  Switch/1 -> Scope1/1, [contacto]
  [contacto] -> Sum/3
  Constant1/1 -> Integrator1/2
  [dxl] -> Gain3/1
  [altura] -> Switch/2
  [altura] -> Switch1/2
  Constant3/1 -> Switch1/3
  Gain3/1 -> Switch1/1
  Switch1/1 -> Sum4/1
  Sum4/1 -> Scope2/1, Divide1/1
  Switch2/1 -> estadoContacto/1
  Constant2/1 -> Switch2/3
  Constant4/1 -> Switch2/1
  [altura] -> Switch2/2
  Constant5/1 -> Integrator3/2

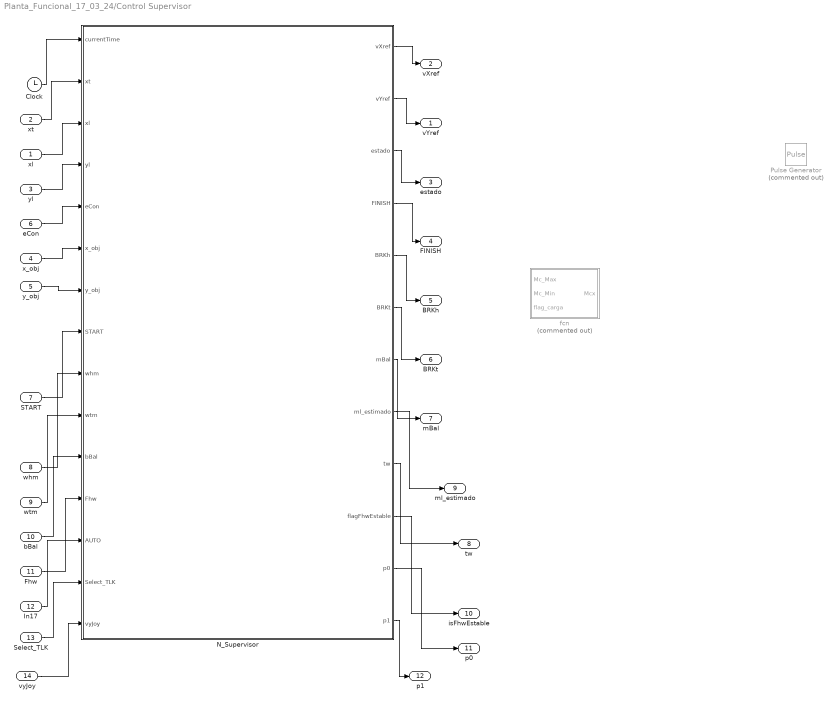
== system Planta_Funcional_17_03_24/Control Supervisor ==
  xl : Inport
  xt : Inport  Port=2
  yl : Inport  Port=3
  x_obj : Inport  Port=4
  y_obj : Inport  Port=5
  eCon : Inport  Port=6
  START : Inport  Port=7
  whm : Inport  Port=8
  wtm : Inport  Port=9
  bBal : Inport  Port=10
  Fhw : Inport  Port=11
  In17 : Inport  Port=12
  Select_TLK : Inport  Port=13
  vyJoy : Inport  Port=14
  Clock : Clock
  N_Supervisor : Stateflow chart  TreatAsAtomicUnit=on
      settings: PortSchema="{\"entries\":[{\"content\":{\"sides\":[{\"content\":{\"connectorIds\":[\"In5\",\"In3\",\"In1\",\"In2\",\"In4\",\"In12\",\"In13\",\"In6\",\"In7\",\"In8\",\"In9\",\"In10\",\"In11\",\"In14\",\"In15\"]},\"type\":\"ConnectorPlacement.EquallySpacedRectSide\",\"uuid\":\"7754e6e1-1487-4c5e-b93c-5b95548dc503\"},{\"content\":{\"connectorIds\":[\"Out1\",\"Out2\",\"Out3\",\"Out4\",\"Out5\",\"Out6\",\"Out7\",\"Out8\",\"Out9\",\"Out10\",\"Out11\",\"Out12\"],\"side\":\"RIGHT\"},\"type\":\"ConnectorPlacement.EquallySpacedRectSide\",\"uuid\":\"e49bdf6e-b30d-4ce2-b56a-406d79434d70\"},{\"content\":{\"connectorIds\":[],\"side\":\"TOP\"},\"type\":\"ConnectorPlacement.EquallySpacedRectSide\",\"uuid\":\"816dde99-88b4-4e51-8e7c-8334ef27840c\"}]},\"type\":\"ConnectorPlacement.EquallySpacedConnector\",\"uuid\":\"e43ca6b0-ace3-4be2-8389-da1b8832a6a4\"}],\"packageUris\":[\"http://schema.mathworks.com/mf0/Connector/R2020b\"],\"version\":\"1.0\"}"
  Pulse Generator : DiscretePulseGenerator  Commented=on  PulseType=Time based  Period=10  PulseWidth=5
  fcn : MATLAB Function  Commented=on  TreatAsAtomicUnit=on
  vYref : Outport
  vXref : Outport  Port=2
  estado : Outport  Port=3
  FINISH : Outport  Port=4
  BRKh : Outport  Port=5
  BRKt : Outport  Port=6
  mBal : Outport  Port=7
  tw : Outport  Port=8
  ml_estimado : Outport  Port=9
  isFhwEstable : Outport  Port=10
  p0 : Outport  Port=11
  p1 : Outport  Port=12
  wires:
  xt/1 -> N_Supervisor/3(xt)
  Fhw/1 -> N_Supervisor/10(Fhw)
  Clock/1 -> N_Supervisor/5(currentTime)
  y_obj/1 -> N_Supervisor/13(y_obj)
  x_obj/1 -> N_Supervisor/12(x_obj)
  N_Supervisor/5(BRKh) -> BRKh/1
  N_Supervisor/1(vXref) -> vXref/1
  N_Supervisor/6(BRKt) -> BRKt/1
  bBal/1 -> N_Supervisor/9(bBal)
  xl/1 -> N_Supervisor/1(xl)
  N_Supervisor/7(mBal) -> mBal/1
  N_Supervisor/3(estado) -> estado/1
  In17/1 -> N_Supervisor/11(AUTO)
  wtm/1 -> N_Supervisor/8(wtm)
  whm/1 -> N_Supervisor/7(whm)
  eCon/1 -> N_Supervisor/4(eCon)
  N_Supervisor/4(FINISH) -> FINISH/1
  START/1 -> N_Supervisor/6(START)
  N_Supervisor/2(vYref) -> vYref/1
  yl/1 -> N_Supervisor/2(yl)
  N_Supervisor/9(tw) -> tw/1
  Select_TLK/1 -> N_Supervisor/14(Select_TLK)
  vyJoy/1 -> N_Supervisor/15(vyJoy)
  N_Supervisor/8(ml_estimado) -> ml_estimado/1
  N_Supervisor/10(flagFhwEstable) -> isFhwEstable/1
  N_Supervisor/11(p0) -> p0/1
  N_Supervisor/12(p1) -> p1/1

== system Planta_Funcional_17_03_24/Controles ==
  Lamp : LampBlock
  Lamp1 : LampBlock
  Lamp2 : LampBlock
  Rocker Switch : RockerSwitchBlock
      settings: Values={{'Off', 'On'}, [0 1]}
  Rocker Switch1 : RockerSwitchBlock
      settings: Values={{'Off', 'On'}, [0 1]}
  Rocker Switch2 : RockerSwitchBlock
      settings: Values={{'Off', 'On'}, [0 1]}

== system Planta_Funcional_17_03_24/Estimacion de Masa ==
  Fhw : Inport
  Constant : Constant  Value=g
  Divide : Product  Inputs=*/
  Gain : Gain  Gain=2
  ml : Outport
  wires:
  Fhw/1 -> Gain/1
  Gain/1 -> Divide/1
  Constant/1 -> Divide/2
  Divide/1 -> ml/1

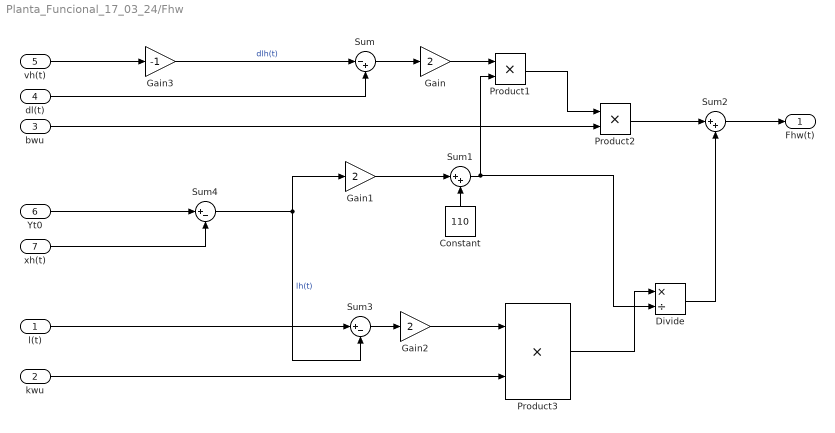
== system Planta_Funcional_17_03_24/Fhw ==
  l(t) : Inport
  kwu : Inport  Port=2
  bwu : Inport  Port=3
  dl(t) : Inport  Port=4
  vh(t) : Inport  Port=5
  Yt0 : Inport  Port=6
  xh(t) : Inport  Port=7
  Constant : Constant  Value=110
  Divide : Product  Inputs=*/
  Gain : Gain  Gain=2
  Gain1 : Gain  Gain=2
  Gain2 : Gain  Gain=2
  Gain3 : Gain  Gain=-1
  Product1 : Product
  Product2 : Product
  Product3 : Product
  Sum : Sum  Inputs=|-+
  Sum1 : Sum  Inputs=|++
  Sum2 : Sum  Inputs=|++
  Sum3 : Sum  Inputs=|+-
  Sum4 : Sum  Inputs=|+-
  Fhw(t) : Outport
  wires:
  dl(t)/1 -> Sum/2
  Sum/1 -> Gain/1
  Gain1/1 -> Sum1/1
  Sum4/1 -> Sum3/2, Gain1/1  "lh(t)"
  l(t)/1 -> Sum3/1
  Constant/1 -> Sum1/2
  Gain/1 -> Product1/1
  Sum1/1 -> Product1/2, Divide/2
  Product1/1 -> Product2/1
  bwu/1 -> Product2/2
  Product2/1 -> Sum2/1
  Sum3/1 -> Gain2/1
  Gain2/1 -> Product3/1
  kwu/1 -> Product3/2
  Product3/1 -> Divide/1
  Divide/1 -> Sum2/2
  Sum2/1 -> Fhw(t)/1
  vh(t)/1 -> Gain3/1
  Gain3/1 -> Sum/1  "dlh(t)"
  Yt0/1 -> Sum4/1
  xh(t)/1 -> Sum4/2

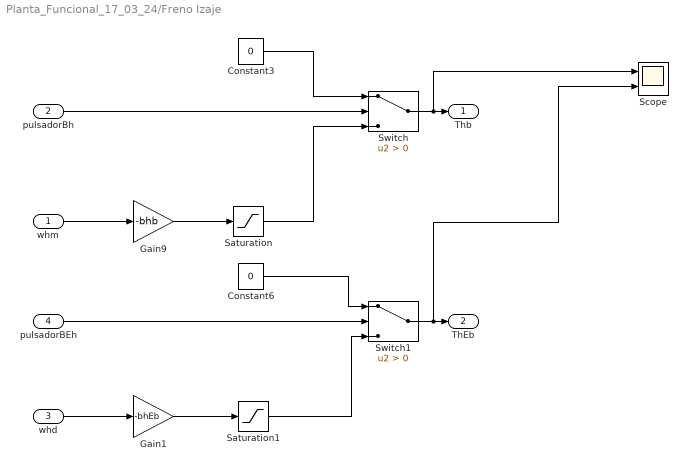
== system Planta_Funcional_17_03_24/Freno Izaje ==
  whm : Inport
  pulsadorBh : Inport  Port=2
  whd : Inport  Port=3
  pulsadorBEh : Inport  Port=4
  Constant3 : Constant  Value=0
  Constant6 : Constant  Value=0
  Gain1 : Gain  Gain=-bhEb
  Gain9 : Gain  Gain=-bhb
  Saturation : Saturate  UpperLimit=Thb_Max  LowerLimit=-Thb_Max
  Saturation1 : Saturate  UpperLimit=ThEb_Max  LowerLimit=-ThEb_Max
  Scope : Scope  NumInputPorts=2
  Switch : Switch  Criteria=u2 > Threshold
  Switch1 : Switch  Criteria=u2 > Threshold
  Thb : Outport  VectorParamsAs1DForOutWhenUnconnected=off
  ThEb : Outport  Port=2  VectorParamsAs1DForOutWhenUnconnected=off
  wires:
  whm/1 -> Gain9/1
  Gain9/1 -> Saturation/1
  Saturation/1 -> Switch/3
  Switch/1 -> Scope/1, Thb/1
  pulsadorBh/1 -> Switch/2
  Constant3/1 -> Switch/1
  pulsadorBEh/1 -> Switch1/2
  Gain1/1 -> Saturation1/1
  Saturation1/1 -> Switch1/3
  Constant6/1 -> Switch1/1
  whd/1 -> Gain1/1
  Switch1/1 -> Scope/2, ThEb/1

== system Planta_Funcional_17_03_24/Freno carro ==
  wtm : Inport
  pulsadorTb : Inport  Port=2
  Constant3 : Constant  Value=0
  Gain9 : Gain  Gain=-btb
  Saturation : Saturate  UpperLimit=Ttb_Max  LowerLimit=-Ttb_Max
  Scope : Scope
  Switch : Switch  Criteria=u2 > Threshold
  Ttb : Outport  VectorParamsAs1DForOutWhenUnconnected=off
  wires:
  wtm/1 -> Gain9/1
  Saturation/1 -> Switch/3
  Switch/1 -> Scope/1, Ttb/1
  pulsadorTb/1 -> Switch/2
  Constant3/1 -> Switch/1
  Gain9/1 -> Saturation/1

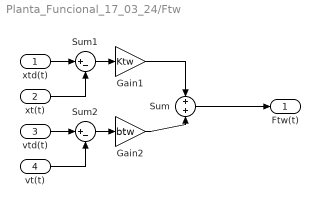
== system Planta_Funcional_17_03_24/Ftw ==
  xtd(t) : Inport
  xt(t) : Inport  Port=2
  vtd(t) : Inport  Port=3
  vt(t) : Inport  Port=4
  Gain1 : Gain  Gain=Ktw
  Gain2 : Gain  Gain=btw
  Sum : Sum
  Sum1 : Sum  Inputs=|+-
  Sum2 : Sum  Inputs=|+-
  Ftw(t) : Outport
  wires:
  Sum2/1 -> Gain2/1
  xtd(t)/1 -> Sum1/1
  vt(t)/1 -> Sum2/2
  xt(t)/1 -> Sum1/2
  Sum/1 -> Ftw(t)/1
  vtd(t)/1 -> Sum2/1
  Gain2/1 -> Sum/2
  Gain1/1 -> Sum/1
  Sum1/1 -> Gain1/1

== system Planta_Funcional_17_03_24/Modulador de Torque Carro ==
  Ttm*(t) : Inport
  Gain1 : Gain  Gain=1/tau_tm
  Integrator : Integrator
  Sum : Sum  Inputs=|+-
  Ttm(t) : Outport
  wires:
  Gain1/1 -> Integrator/1
  Integrator/1 -> Ttm(t)/1, Sum/2
  Ttm*(t)/1 -> Sum/1
  Sum/1 -> Gain1/1

== system Planta_Funcional_17_03_24/Modulador de Torque Izaje ==
  Thm*(t) : Inport
  Gain1 : Gain  Gain=1/tau_hm
  Integrator : Integrator
  Sum : Sum  Inputs=|+-
  Thm(t) : Outport
  wires:
  Gain1/1 -> Integrator/1
  Integrator/1 -> Thm(t)/1, Sum/2
  Thm*(t)/1 -> Sum/1
  Sum/1 -> Gain1/1

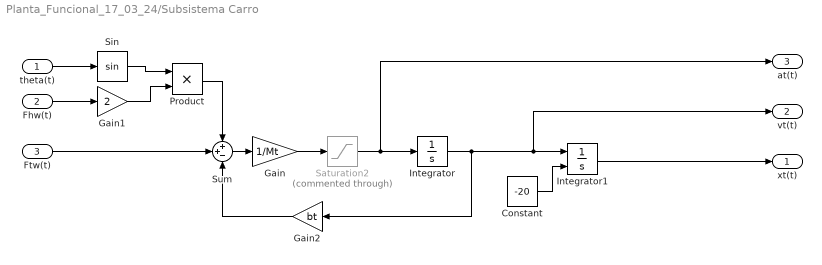
== system Planta_Funcional_17_03_24/Subsistema Carro ==
  theta(t) : Inport
  Fhw(t) : Inport  Port=2
  Ftw(t) : Inport  Port=3
  Constant : Constant  Value=-20
  Gain : Gain  Gain=1/Mt
  Gain1 : Gain  Gain=2
  Gain2 : Gain  Gain=bt
  Integrator : Integrator
  Integrator1 : Integrator  InitialConditionSource=external
  Product : Product
  Saturation2 : Saturate  Commented=through  UpperLimit=atmax  LowerLimit=-atmax
  Sin : Trigonometry
  Sum : Sum  Inputs=++-
  xt(t) : Outport
  vt(t) : Outport  Port=2
  at(t) : Outport  Port=3
  wires:
  Integrator/1 -> vt(t)/1, Integrator1/1, Gain2/1
  Gain1/1 -> Product/2
  theta(t)/1 -> Sin/1
  Sum/1 -> Gain/1
  Product/1 -> Sum/1
  Integrator1/1 -> xt(t)/1
  Ftw(t)/1 -> Sum/2
  Gain2/1 -> Sum/3
  Fhw(t)/1 -> Gain1/1
  Sin/1 -> Product/1
  Gain/1 -> Saturation2/1
  Constant/1 -> Integrator1/2
  Saturation2/1 -> at(t)/1, Integrator/1

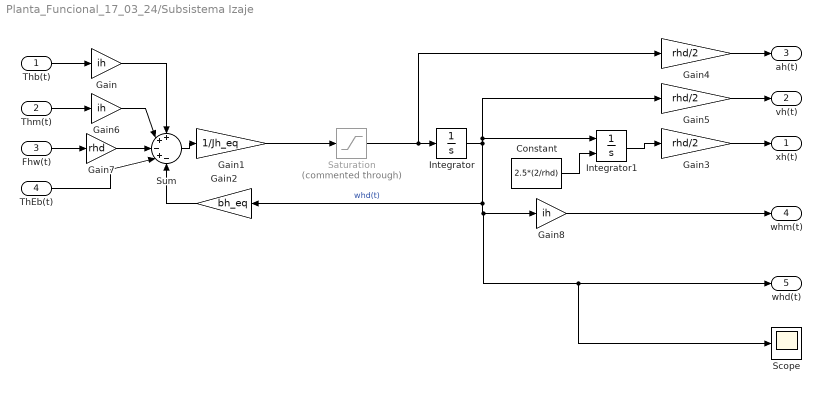
== system Planta_Funcional_17_03_24/Subsistema Izaje ==
  Thb(t) : Inport
  Thm(t) : Inport  Port=2
  Fhw(t) : Inport  Port=3
  ThEb(t) : Inport  Port=4
  Constant : Constant  Value=2.5*(2/rhd)
  Gain : Gain  Gain=ih
  Gain1 : Gain  Gain=1/Jh_eq
  Gain2 : Gain  Gain=bh_eq
  Gain3 : Gain  Gain=rhd/2
  Gain4 : Gain  Gain=rhd/2
  Gain5 : Gain  Gain=rhd/2
  Gain6 : Gain  Gain=ih
  Gain7 : Gain  Gain=rhd
  Gain8 : Gain  Gain=ih
  Integrator : Integrator
  Integrator1 : Integrator  InitialConditionSource=external
  Saturation : Saturate  Commented=through  UpperLimit=alfahmax  LowerLimit=-alfahmax
  Scope : Scope
  Sum : Sum  Inputs=++-+-
  xh(t) : Outport
  vh(t) : Outport  Port=2
  ah(t) : Outport  Port=3
  whm(t) : Outport  Port=4
  whd(t) : Outport  Port=5
  wires:
  Integrator/1 -> Gain5/1, Integrator1/1, Scope/1, whd(t)/1, Gain8/1, Gain2/1  "whd(t)"
  Gain2/1 -> Sum/5
  Gain4/1 -> ah(t)/1
  Gain3/1 -> xh(t)/1
  Gain5/1 -> vh(t)/1
  Fhw(t)/1 -> Gain7/1
  Integrator1/1 -> Gain3/1
  Thb(t)/1 -> Gain/1
  Gain1/1 -> Saturation/1
  Sum/1 -> Gain1/1
  Thm(t)/1 -> Gain6/1
  Gain/1 -> Sum/1
  Gain6/1 -> Sum/2
  Gain7/1 -> Sum/3
  ThEb(t)/1 -> Sum/4
  Gain8/1 -> whm(t)/1
  Constant/1 -> Integrator1/2
  Saturation/1 -> Gain4/1, Integrator/1

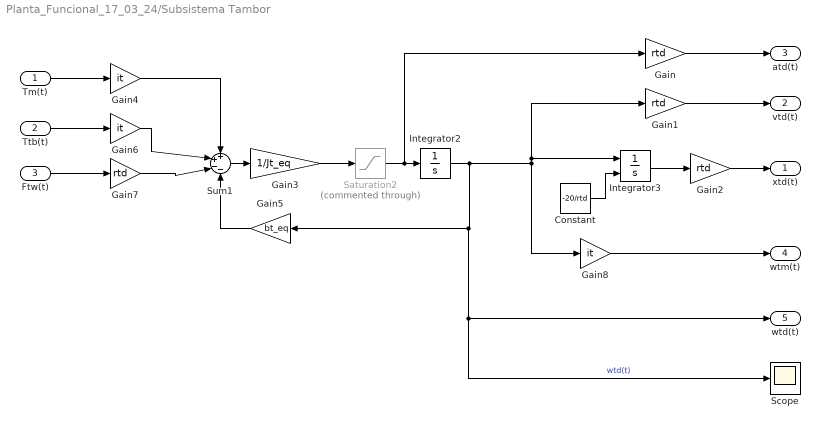
== system Planta_Funcional_17_03_24/Subsistema Tambor ==
  Tm(t) : Inport
  Ttb(t) : Inport  Port=2
  Ftw(t) : Inport  Port=3
  Constant : Constant  Value=-20/rtd
  Gain{,1..2,7} (4 alike) : Gain  Gain=rtd
  Gain3 : Gain  Gain=1/Jt_eq
  Gain4 : Gain  Gain=it
  Gain5 : Gain  Gain=bt_eq
  Gain6 : Gain  Gain=it
  Gain8 : Gain  Gain=it
  Integrator2 : Integrator
  Integrator3 : Integrator  InitialConditionSource=external
  Saturation2 : Saturate  Commented=through  UpperLimit=alfatmax  LowerLimit=-alfatmax
  Scope : Scope
  Sum1 : Sum  Inputs=++--
  xtd(t) : Outport
  vtd(t) : Outport  Port=2
  atd(t) : Outport  Port=3
  wtm(t) : Outport  Port=4
  wtd(t) : Outport  Port=5
  wires:
  Integrator3/1 -> Gain2/1
  Ftw(t)/1 -> Gain7/1
  Gain2/1 -> xtd(t)/1
  Integrator2/1 -> Gain1/1, Integrator3/1, Gain8/1, Scope/1, wtd(t)/1, Gain5/1  "wtd(t)"
  Tm(t)/1 -> Gain4/1
  Ttb(t)/1 -> Gain6/1
  Sum1/1 -> Gain3/1
  Gain5/1 -> Sum1/4
  Gain1/1 -> vtd(t)/1
  Gain/1 -> atd(t)/1
  Gain4/1 -> Sum1/1
  Gain6/1 -> Sum1/2
  Gain7/1 -> Sum1/3
  Gain8/1 -> wtm(t)/1
  Gain3/1 -> Saturation2/1
  Constant/1 -> Integrator3/2
  Saturation2/1 -> Gain/1, Integrator2/1

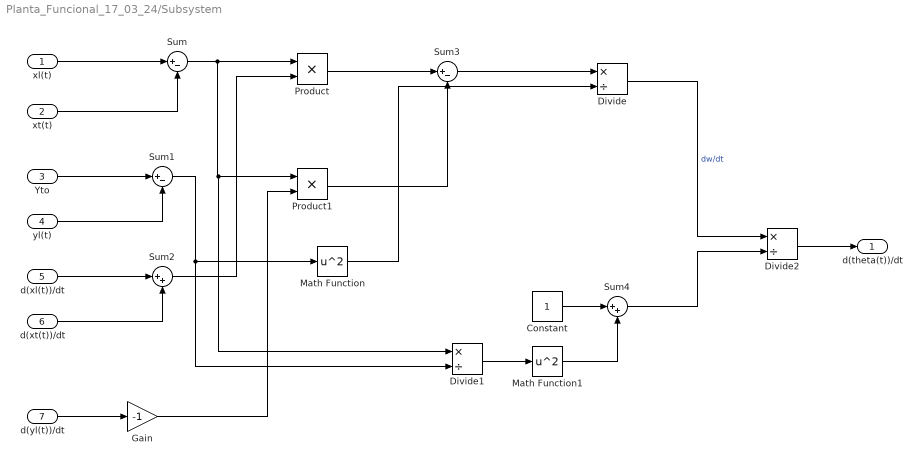
== system Planta_Funcional_17_03_24/Subsystem ==
  xl(t) : Inport
  xt(t) : Inport  Port=2
  Yto : Inport  Port=3
  yl(t) : Inport  Port=4
  d(xl(t))/dt : Inport  Port=5
  d(xt(t))/dt : Inport  Port=6
  d(yl(t))/dt : Inport  Port=7
  Constant : Constant
  Divide : Product  Inputs=*/
  Divide1 : Product  Inputs=*/
  Divide2 : Product  Inputs=*/
  Gain : Gain  Gain=-1
  Math Function : Math  Operator=square  SaturateOnIntegerOverflow=on
  Math Function1 : Math  Operator=square  SaturateOnIntegerOverflow=on
  Product : Product
  Product1 : Product
  Sum : Sum  Inputs=|+-
  Sum1 : Sum  Inputs=|+-
  Sum2 : Sum  Inputs=|++
  Sum3 : Sum  Inputs=|+-
  Sum4 : Sum  Inputs=|++
  d(theta(t))/dt : Outport
  wires:
  xl(t)/1 -> Sum/1
  xt(t)/1 -> Sum/2
  Yto/1 -> Sum1/1
  yl(t)/1 -> Sum1/2
  Sum/1 -> Divide1/1, Product1/1, Product/1
  d(xl(t))/dt/1 -> Sum2/1
  d(xt(t))/dt/1 -> Sum2/2
  Sum2/1 -> Product/2
  Product/1 -> Sum3/1
  Product1/1 -> Sum3/2
  d(yl(t))/dt/1 -> Gain/1
  Gain/1 -> Product1/2
  Sum3/1 -> Divide/1
  Sum1/1 -> Math Function/1, Divide1/2
  Math Function/1 -> Divide/2
  Divide/1 -> Divide2/1  "dw/dt"
  Divide1/1 -> Math Function1/1
  Math Function1/1 -> Sum4/2
  Constant/1 -> Sum4/1
  Divide2/1 -> d(theta(t))/dt/1
  Sum4/1 -> Divide2/2
